simulink library "Median_Filter_5th_lib"  (R2022a)
settings: Solver=VariableStepAuto  StartTime=0.0  StopTime=10.0  RelTol=1e-3
settings Model: Creator=FAbdelkarim  LastModifiedBy=FAbdelkarim

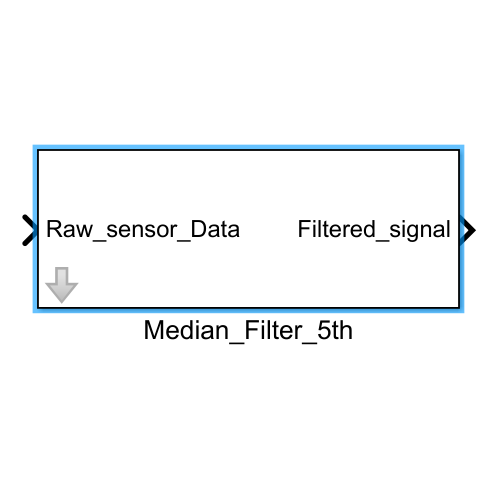
[thumbnail: Simulink's stored preview of the top-level diagram]
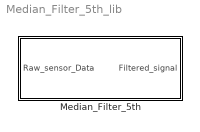
== system Median_Filter_5th_lib ==
  Median_Filter_5th : Subsystem
      mask DialogControl MedianFilter Prompt: (Median Filter)

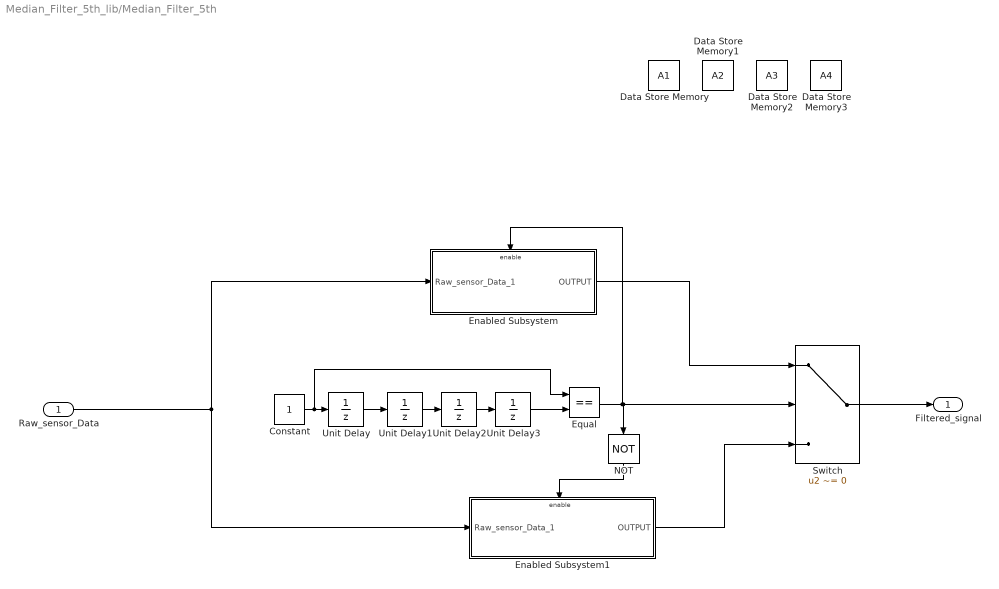
== system Median_Filter_5th_lib/Median_Filter_5th ==
  Raw_sensor_Data : Inport
  Constant : Constant  SampleTime=-1
  Data Store Memory : DataStoreMemory  DataStoreName=A1  WriteAfterWriteMsg=warning  ShowAdditionalParam=off
  Data Store Memory1 : DataStoreMemory  DataStoreName=A2  WriteAfterWriteMsg=warning  ShowAdditionalParam=off
  Data Store Memory2 : DataStoreMemory  DataStoreName=A3  WriteAfterWriteMsg=warning  ShowAdditionalParam=off
  Data Store Memory3 : DataStoreMemory  DataStoreName=A4  WriteAfterWriteMsg=warning  ShowAdditionalParam=off
  Enabled Subsystem : Subsystem  TreatAsAtomicUnit=on
  Enabled Subsystem1 : Subsystem  TreatAsAtomicUnit=on
  Equal : RelationalOperator  Operator===  OutDataTypeStr=boolean  RndMeth=Simplest  InputSameDT=off
  NOT : Logic  Operator=NOT  IconShape=distinctive  AllPortsSameDT=off  OutDataTypeStr=boolean
  Switch : Switch  Criteria=u2 ~= 0  SaturateOnIntegerOverflow=off  InputSameDT=off
  Unit Delay{,1..3} (4 alike) : UnitDelay  SampleTime=-1  HasFrameUpgradeWarning=on
  Filtered_signal : Outport
  wires:
  NOT/1 -> Enabled Subsystem1/Enable
  Unit Delay3/1 -> Equal/2
  Constant/1 -> Equal/1, Unit Delay/1
  Unit Delay/1 -> Unit Delay1/1
  Equal/1 -> Switch/2, NOT/1, Enabled Subsystem/Enable
  Enabled Subsystem1/1(OUTPUT) -> Switch/3
  Unit Delay2/1 -> Unit Delay3/1
  Unit Delay1/1 -> Unit Delay2/1
  Enabled Subsystem/1(OUTPUT) -> Switch/1
  Raw_sensor_Data/1 -> Enabled Subsystem/1(Raw_sensor_Data_1), Enabled Subsystem1/1(Raw_sensor_Data_1)
  Switch/1 -> Filtered_signal/1

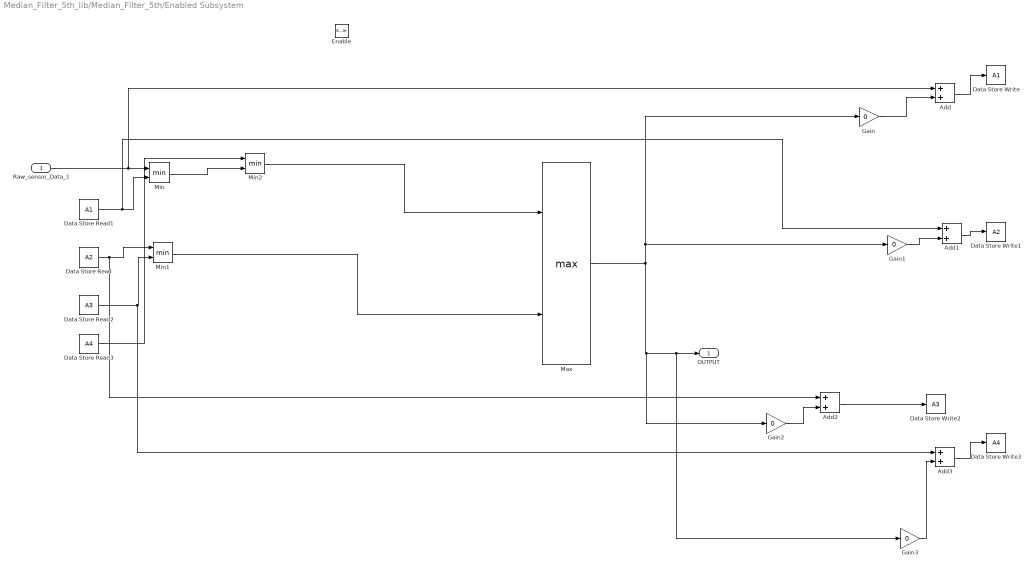
== system Median_Filter_5th_lib/Median_Filter_5th/Enabled Subsystem ==
  Raw_sensor_Data_1 : Inport
  Enable : EnablePort
  Add{,1..3} (4 alike) : Sum
  Data Store Read : DataStoreRead  DataStoreName=A2  IndexOptions=Index vector (dialog)  Indices=1  OutputSizes=1
  Data Store Read1 : DataStoreRead  DataStoreName=A1  IndexOptions=Index vector (dialog)  Indices=1  OutputSizes=1
  Data Store Read2 : DataStoreRead  DataStoreName=A3  IndexOptions=Index vector (dialog)  Indices=1  OutputSizes=1
  Data Store Read3 : DataStoreRead  DataStoreName=A4  IndexOptions=Index vector (dialog)  Indices=1  OutputSizes=1
  Data Store Write : DataStoreWrite  DataStoreName=A1  IndexOptions=Index vector (dialog)  Indices=1  OutputSizes=1
  Data Store Write1 : DataStoreWrite  DataStoreName=A2  IndexOptions=Index vector (dialog)  Indices=1  OutputSizes=1
  Data Store Write2 : DataStoreWrite  DataStoreName=A3  IndexOptions=Index vector (dialog)  Indices=1  OutputSizes=1
  Data Store Write3 : DataStoreWrite  DataStoreName=A4  IndexOptions=Index vector (dialog)  Indices=1  OutputSizes=1
  Gain{,1..3} (4 alike) : Gain  Gain=0
  Max : MinMax  Function=max  Inputs=2
  Min : MinMax  Inputs=2
  Min1 : MinMax  Inputs=2
  Min2 : MinMax  Inputs=2
  OUTPUT : Outport
  wires:
  Max/1 -> Gain1/1, Gain/1, Gain2/1, Gain3/1, OUTPUT/1
  Raw_sensor_Data_1/1 -> Add/1, Min/1
  Data Store Read1/1 -> Add1/1, Min/2
  Data Store Read/1 -> Add2/1, Min1/1
  Data Store Read2/1 -> Add3/1, Min1/2
  Data Store Read3/1 -> Min2/1
  Min/1 -> Min2/2
  Min2/1 -> Max/1
  Min1/1 -> Max/2
  Add/1 -> Data Store Write/1
  Gain/1 -> Add/2
  Gain1/1 -> Add1/2
  Add1/1 -> Data Store Write1/1
  Gain2/1 -> Add2/2
  Add2/1 -> Data Store Write2/1
  Gain3/1 -> Add3/2
  Add3/1 -> Data Store Write3/1

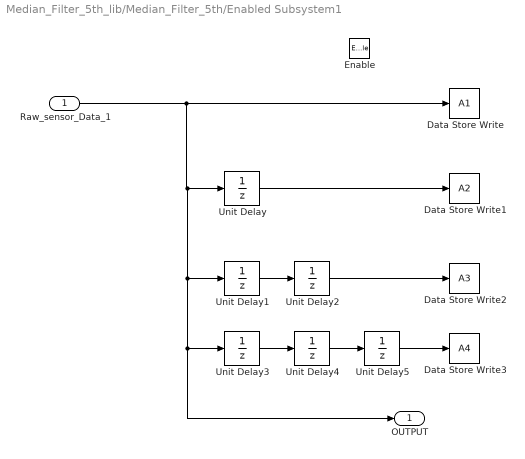
== system Median_Filter_5th_lib/Median_Filter_5th/Enabled Subsystem1 ==
  Raw_sensor_Data_1 : Inport
  Enable : EnablePort
  Data Store Write : DataStoreWrite  DataStoreName=A1  IndexOptions=Index vector (dialog)  Indices=1  OutputSizes=1
  Data Store Write1 : DataStoreWrite  DataStoreName=A2  IndexOptions=Index vector (dialog)  Indices=1  OutputSizes=1
  Data Store Write2 : DataStoreWrite  DataStoreName=A3  IndexOptions=Index vector (dialog)  Indices=1  OutputSizes=1
  Data Store Write3 : DataStoreWrite  DataStoreName=A4  IndexOptions=Index vector (dialog)  Indices=1  OutputSizes=1
  Unit Delay{,1..5} (6 alike) : UnitDelay  SampleTime=-1  HasFrameUpgradeWarning=on
  OUTPUT : Outport
  wires:
  Raw_sensor_Data_1/1 -> OUTPUT/1, Unit Delay3/1, Unit Delay1/1, Unit Delay/1, Data Store Write/1
  Unit Delay5/1 -> Data Store Write3/1
  Unit Delay4/1 -> Unit Delay5/1
  Unit Delay1/1 -> Unit Delay2/1
  Unit Delay3/1 -> Unit Delay4/1
  Unit Delay/1 -> Data Store Write1/1
  Unit Delay2/1 -> Data Store Write2/1
